simulink model "ForceField_Reaching"  (R2023b)
settings: Solver=FixedStepDiscrete  StartTime=0.0  StopTime=inf  FixedStep=0.001  RelTol=1e-3
libraries: PhanTorque_3Dof_Library_64Bits x2, vrlib x2, simulink x1
settings Model: Creator=carlos.aldana  LastModifiedBy=galvd
settings SolverCC: AlgebraicLoopSolver=TrustRegion
settings DataIOCC: LimitDataPoints=on  SaveFormat=Array  ReturnWorkspaceOutputs=off
settings OptimizationCC: BlockReduction=off  BooleanDataType=off  ReuseModelBlockBuffer=off  LifeSpan=inf
settings DebuggingCC: SaveWithParameterizedLinksMsg=none  UnderspecifiedInitializationDetection=Classic  MergeDetectMultiDrivingBlocksExec=none  SignalResolutionControl=TryResolveAllWithWarning  UnconnectedInputMsg=warning  UnconnectedOutputMsg=warning  UnconnectedLineMsg=warning  AllowSymbolicDim=off  SFUnexpectedBacktrackingDiag=warning  SFNoUnconditionalDefaultTransitionDiag=warning  SFExecutionAtInitializationDiag=none  ArithmeticOperatorsInVariantConditions=warning
settings HardwareCC: ProdBitPerPointer=32  ProdBitPerSizeT=32  ProdBitPerPtrDiffT=32  ProdLargestAtomicFloat=None  ProdIntDivRoundTo=Undefined  ProdEndianess=Unspecified  ProdWordSize=32  ProdHWDeviceType=32-bit Generic  TargetUnknown=on
settings ModelReferenceCC: EnableRefExpFcnMdlSchedulingChecks=on  PropagateSignalLabelsOutOfModel=off
settings SFSimCC: SimUseLocalCustomCode=off  CustomCodeUndefinedFunction=UseInterfaceOnly
settings RTWCC: RTWUseLocalCustomCode=off  DLArmComputeVersion=19.05
settings CodeAppCC: StateflowObjectComments=on
settings GRTTargetCC: TargetLangStandard=C89/C90 (ANSI)
settings ConfigComp: CovMetricSettings=dw  CovSaveCumulativeToWorkspaceVar=on  CovSaveSingleToWorkspaceVar=on  CovExternalEMLEnable=off  CovSFcnEnable=off

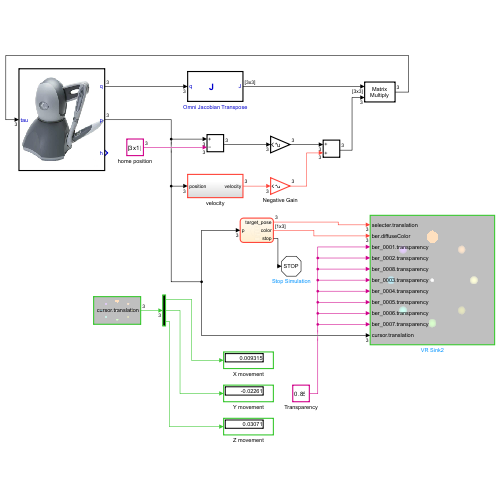
[thumbnail: Simulink's stored preview of the top-level diagram]
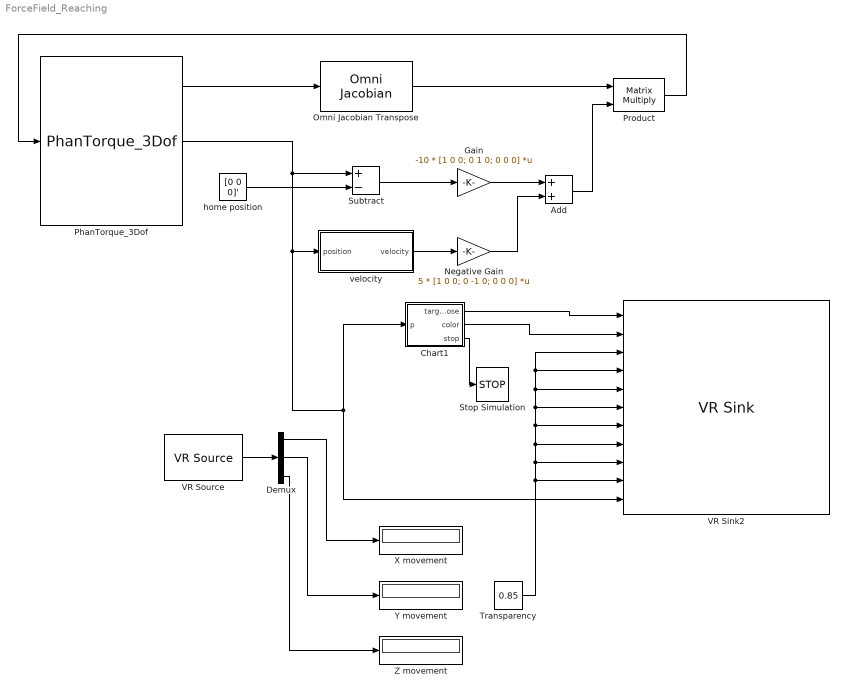
== system ForceField_Reaching ==
  Add : Sum
  Chart1 : Stateflow chart  TreatAsAtomicUnit=on
  Demux : Demux  Outputs=3
  Gain : Gain  Gain=-10 * [1 0 0; 0 1 0; 0 0 0]  Multiplication=Matrix(K*u)
  Negative Gain : Gain  Gain=5 * [1 0 0; 0 -1 0; 0 0 0]  Multiplication=Matrix(K*u)
  Omni Jacobian Transpose : PhanTorque_3Dof_Library_64Bits/Omni Jacobian  SystemSampleTime=-1  VariantActivationTime=update diagram  AllowFlexibleInterface=on  Latency=0  AutoFrameSizeCalculation=off
      link override MATLAB Fcn: MATLABFcn=Omni_Jacobian_Transpose(u)
  PhanTorque_3Dof : PhanTorque_3Dof_Library_64Bits/PhanTorque_3Dof  Haptic_Name='Default Device'
  Product : Product  Multiplication=Matrix(*)
  Stop Simulation : Stop
  Subtract : Sum  Inputs=+-
  Transparency : Constant  Value=0.85
  VR Sink2 : vrlib/VR Sink  InstantiateOnLoad=on  SampleTime=0.1  ViewEnable=on  RemoteChange=off  RemoteView=off  FieldsWritten=selecter.translation.3.1.1.double#ber.diffuseColor.3.1.1.double#ber_0001.transparency.1.1.1.double#ber_0002.transparency.1.1.1.double#ber_0008.transparency.1.1.1.double#ber_0003.transparency.1.1.1.double#ber_0004.transparency.1.1.1.double#ber_0005.transparency.1.1.1.double#ber_0006.transparency.1.1.1.double#ber_0007.transparency.1.1.1.double#cursor.translation.3.1.1.double  WorldFileName=8_palline_color.wrl  AutoView=off  VideoDimensions=[]  AllowVariableSize=off
  VR Source : vrlib/VR Source  InstantiateOnLoad=on  SampleTime=0.1  ViewEnable=on  RemoteChange=off  RemoteView=off  FieldsRead=cursor.translation.1.3.1.double  WorldFileName=8_palline_color.wrl  AutoView=off  VideoDimensions=[]  AllowVariableSize=off
  X movement : Display
  Y movement : Display
  Z movement : Display
  home position : Constant  Value=[0 0 0]'
  velocity : Subsystem
  wires:
  home position/1 -> Subtract/2
  PhanTorque_3Dof/1 -> Omni Jacobian Transpose/1
  Gain/1 -> Add/1
  Negative Gain/1 -> Add/2
  Omni Jacobian Transpose/1 -> Product/1
  Product/1 -> PhanTorque_3Dof/1
  Subtract/1 -> Gain/1
  velocity/1(velocity) -> Negative Gain/1
  Add/1 -> Product/2
  Demux/1 -> X movement/1
  Chart1/2(color) -> VR Sink2/2
  PhanTorque_3Dof/2 -> velocity/1(position), VR Sink2/11, Chart1/1(p), Subtract/1
  VR Source/1 -> Demux/1
  Transparency/1 -> VR Sink2/5, VR Sink2/3, VR Sink2/4, VR Sink2/6, VR Sink2/7, VR Sink2/8, VR Sink2/9, VR Sink2/10
  Chart1/1(target_pose) -> VR Sink2/1
  Demux/2 -> Y movement/1
  Demux/3 -> Z movement/1
  Chart1/3(stop) -> Stop Simulation/1

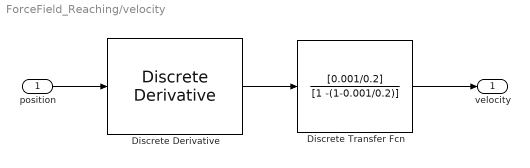
== system ForceField_Reaching/velocity ==
  position : Inport
  Discrete Derivative : simulink/Discrete/Discrete Derivative  gainval=1.0  ICPrevScaledInput=0.0  OutMin=[]  OutMax=[]  OutDataType=fixdt(1, 16)  OutScaling=2^-10  DoSatur=off
  Discrete Transfer Fcn : DiscreteTransferFcn  Numerator=[0.001/0.2]  Denominator=[1 -(1-0.001/0.2)]
  velocity : Outport  VectorParamsAs1DForOutWhenUnconnected=off
  wires:
  position/1 -> Discrete Derivative/1
  Discrete Derivative/1 -> Discrete Transfer Fcn/1
  Discrete Transfer Fcn/1 -> velocity/1

== stateflow chart ForceField_Reaching/Chart1 ==
  state initial
    entry:
    stop = 0;
    radius=0.1;
    counter=0;
    angle_matrix=[0 pi/4 pi/2 3/4*pi pi 5/4*pi 3/2*pi 7/4*pi];
    % Ensure that each unique angle is included at least once and adding two other angles taken randomly
    random_angles = [angle_matrix(randperm(length(angle_matrix), 8)) angle_matrix(randi(8)) angle_matrix(randi(8))];
  state rand_angle
    angle = random_angles(counter+1);
  state new_target
    entry:
    color=[1 0 0];
    target_pose=radius*[cos(angle); sin(angle); 0];
    err=norm(p(1:2)-target_pose(1:2));
    during:
    err=norm(p(1:2)-target_pose(1:2));
  state feedback
    entry:
    color=[0 0 1];
    during:
    err=norm(p(1:2)-target_pose(1:2));
  state back
    entry:
    target_pose=[0 0 0]';
    color=[1 0 0];
    during:
    err=norm(p(1:2)-target_pose(1:2));
  state feedback2
    entry:
    color=[0 0 1];
    during:
    err=norm(p(1:2)-target_pose(1:2));
  state finish
    stop = 1;
    end
  (default) -> initial
  initial -> rand_angle
  feedback2 -> rand_angle [order 1] : [err<0.01 & after (2, sec) & counter<10]
  rand_angle -> new_target
  feedback -> new_target [order 2] : [err>=0.01]
  new_target -> feedback : [err<0.01]
  feedback -> back [order 1] : [err<0.01 & after(1, sec)]{counter = counter+1;}
  feedback2 -> back [order 2] : [err>=0.01]
  back -> feedback2 : [err<0.01]
  feedback2 -> finish [order 3] : [counter>=10]
  data: p input; target_pose output; color output; angle_matrix local; angle local; counter local; err local; radius local; random_angles local; stop output
